simulink model "SensorModel"  (R2026b)
settings: Solver=ode45  StopTime=Simulation.StopTimeSmoke.Value
undefined symbols (not defined in the file): DefaultSensorBus
settings Model: DataDictionary=VehicleData.sldd  Creator=Xu Dingyi  LastModifiedBy=29358

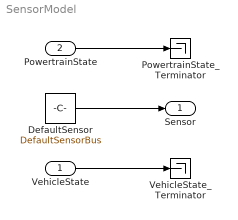
== system SensorModel ==
  VehicleState : Inport  OutDataTypeStr=Bus: VehicleStateBus
  PowertrainState : Inport  Port=2  OutDataTypeStr=Bus: PowertrainStateBus
  DefaultSensor : Constant  Value=DefaultSensorBus  OutDataTypeStr=Bus: SensorBus  SampleTime=-1
  PowertrainState_Terminator : Terminator
  VehicleState_Terminator : Terminator
  Sensor : Outport  OutDataTypeStr=Bus: SensorBus
  wires:
  DefaultSensor/1 -> Sensor/1
  PowertrainState/1 -> PowertrainState_Terminator/1
  VehicleState/1 -> VehicleState_Terminator/1
